simulink library "vehicle_model"  (R2020b)
settings: Solver=ode45  StartTime=0.0  StopTime=10.0  RelTol=1e-3  EnableMultiTasking=on
undefined symbols (not defined in the file): DiscIntNeverNeededParam, par_VEH, select_To_Wks_akt, stepsize, v0
libraries: $bdroot x8, pacejka_trans x6, simulink x4, body_chassis_vert x1
(part 4 of 4)

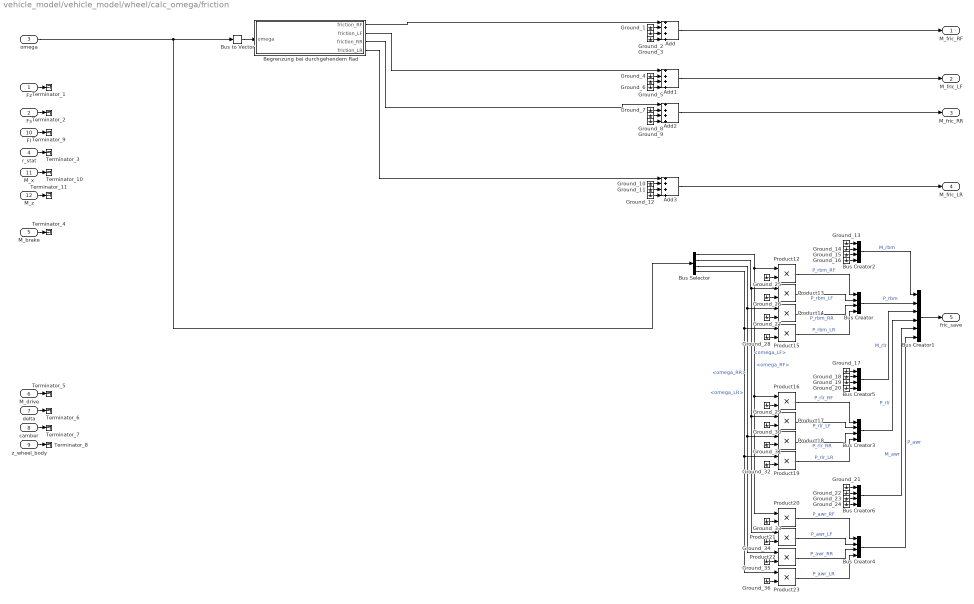
== system vehicle_model/vehicle_model/wheel/calc_omega/friction ==
  Fz : Inport
  Fs : Inport  Port=2
  omega : Inport  Port=3
  r_stat : Inport  Port=4
  M_brake : Inport  Port=5
  M_drive : Inport  Port=6
  delta : Inport  Port=7
  camber : Inport  Port=8
  z_wheel_body : Inport  Port=9
  Fl : Inport  Port=10
  M_x : Inport  Port=11
  M_z : Inport  Port=12
  Add{,1..3} (4 alike) : Sum  Inputs=++++
  Begrenzung bei durchgehendem Rad : Subsystem
  Bus Creator{,2..6} (6 alike) : BusCreator  Inputs=4
  Bus Creator1 : BusCreator  Inputs=6
  Bus Selector : BusSelector  OutputSignals=omega_RF,omega_LF,omega_RR,omega_LR
  Bus to Vector : BusToVector
  Ground_{1..36} (36 alike) : Ground
  Product{12..23} (12 alike) : Product
  Terminator_{1..11} (11 alike) : Terminator
  M_fric_RF : Outport  VectorParamsAs1DForOutWhenUnconnected=off
  M_fric_LF : Outport  Port=2  VectorParamsAs1DForOutWhenUnconnected=off
  M_fric_RR : Outport  Port=3  VectorParamsAs1DForOutWhenUnconnected=off
  M_fric_LR : Outport  Port=4  VectorParamsAs1DForOutWhenUnconnected=off
  fric_save : Outport  Port=5  VectorParamsAs1DForOutWhenUnconnected=off
  wires:
  Ground_36/1 -> Product23/2
  Ground_35/1 -> Product22/2
  Ground_34/1 -> Product21/2
  Ground_33/1 -> Product20/2
  Ground_32/1 -> Product19/2
  Ground_31/1 -> Product18/2
  Ground_30/1 -> Product17/2
  Ground_29/1 -> Product16/2
  Ground_28/1 -> Product15/2
  Ground_27/1 -> Product14/2
  Ground_26/1 -> Product13/2
  Ground_25/1 -> Product12/2
  Ground_24/1 -> Bus Creator6/4
  Ground_23/1 -> Bus Creator6/3
  Ground_22/1 -> Bus Creator6/2
  Ground_21/1 -> Bus Creator6/1
  Ground_20/1 -> Bus Creator5/4
  Ground_19/1 -> Bus Creator5/3
  Ground_18/1 -> Bus Creator5/2
  Ground_17/1 -> Bus Creator5/1
  Ground_16/1 -> Bus Creator2/4
  Ground_15/1 -> Bus Creator2/3
  Ground_14/1 -> Bus Creator2/2
  Ground_13/1 -> Bus Creator2/1
  Ground_12/1 -> Add3/4
  Ground_11/1 -> Add3/3
  Ground_10/1 -> Add3/2
  Ground_9/1 -> Add2/4
  Ground_8/1 -> Add2/3
  Ground_7/1 -> Add2/2
  Ground_6/1 -> Add1/4
  Ground_5/1 -> Add1/3
  Ground_4/1 -> Add1/2
  Ground_3/1 -> Add/4
  Ground_2/1 -> Add/3
  Ground_1/1 -> Add/2
  M_z/1 -> Terminator_11/1
  M_x/1 -> Terminator_10/1
  Fl/1 -> Terminator_9/1
  z_wheel_body/1 -> Terminator_8/1
  camber/1 -> Terminator_7/1
  delta/1 -> Terminator_6/1
  M_drive/1 -> Terminator_5/1
  M_brake/1 -> Terminator_4/1
  r_stat/1 -> Terminator_3/1
  Fs/1 -> Terminator_2/1
  Fz/1 -> Terminator_1/1
  Bus to Vector/1 -> Begrenzung bei durchgehendem Rad/1(omega)
  omega/1 -> Bus Selector/1, Bus to Vector/1
  Begrenzung bei durchgehendem Rad/1(friction_RF) -> Add/1
  Begrenzung bei durchgehendem Rad/2(friction_LF) -> Add1/1
  Begrenzung bei durchgehendem Rad/3(friction_RR) -> Add2/1
  Begrenzung bei durchgehendem Rad/4(friction_LR) -> Add3/1
  Add/1 -> M_fric_RF/1
  Add1/1 -> M_fric_LF/1
  Add2/1 -> M_fric_RR/1
  Add3/1 -> M_fric_LR/1
  Bus Selector/1 -> Product12/1, Product20/1, Product16/1  "<omega_RF>"
  Bus Selector/2 -> Product21/1, Product17/1, Product13/1  "<omega_LF>"
  Bus Selector/3 -> Product22/1, Product18/1, Product14/1  "<omega_RR>"
  Bus Selector/4 -> Product23/1, Product19/1, Product15/1  "<omega_LR>"
  Product12/1 -> Bus Creator/1  "P_rbm_RF"
  Product13/1 -> Bus Creator/2  "P_rbm_LF"
  Product14/1 -> Bus Creator/3  "P_rbm_RR"
  Product15/1 -> Bus Creator/4  "P_rbm_LR"
  Bus Creator/1 -> Bus Creator1/2  "P_rbm"
  Bus Creator2/1 -> Bus Creator1/1  "M_rbm"
  Bus Creator1/1 -> fric_save/1
  Product16/1 -> Bus Creator3/1  "P_rlr_RF"
  Product17/1 -> Bus Creator3/2  "P_rlr_LF"
  Product18/1 -> Bus Creator3/3  "P_rlr_RR"
  Product19/1 -> Bus Creator3/4  "P_rlr_LR"
  Bus Creator5/1 -> Bus Creator1/3  "M_rlr"
  Bus Creator3/1 -> Bus Creator1/4  "P_rlr"
  Product20/1 -> Bus Creator4/1  "P_awr_RF"
  Product21/1 -> Bus Creator4/2  "P_awr_LF"
  Product22/1 -> Bus Creator4/3  "P_awr_RR"
  Product23/1 -> Bus Creator4/4  "P_awr_LR"
  Bus Creator6/1 -> Bus Creator1/5  "M_awr"
  Bus Creator4/1 -> Bus Creator1/6  "P_awr"

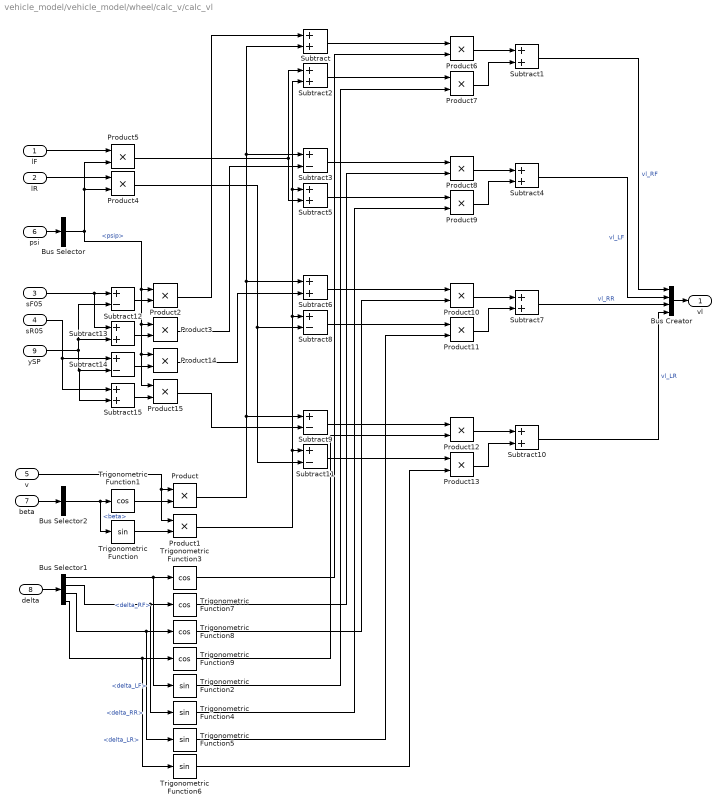
== system vehicle_model/vehicle_model/wheel/calc_v/calc_vl ==
  lF : Inport
  lR : Inport  Port=2
  sF05 : Inport  Port=3
  sR05 : Inport  Port=4
  v : Inport  Port=5
  psi : Inport  Port=6
  beta : Inport  Port=7
  delta : Inport  Port=8
  ySP : Inport  Port=9
  Bus Creator : BusCreator  Inputs=4
  Bus Selector : BusSelector  OutputSignals=psip
  Bus Selector1 : BusSelector  OutputSignals=delta_RF,delta_LF,delta_RR,delta_LR
  Bus Selector2 : BusSelector  OutputSignals=beta
  Product{,1..15} (16 alike) : Product  RndMeth=Zero
  Subtract{,1..2,4..7,10,13,15} (10 alike) : Sum
  Subtract{3,8..9,11..12,14} (6 alike) : Sum  Inputs=+-
  Trigonometric Function{,2,4..6} (5 alike) : Trigonometry
  Trigonometric Function{1,3,7..9} (5 alike) : Trigonometry  Operator=cos
  vl : Outport  VectorParamsAs1DForOutWhenUnconnected=off
  wires:
  Subtract1/1 -> Bus Creator/1  "vl_RF"
  Subtract4/1 -> Bus Creator/2  "vl_LF"
  Subtract7/1 -> Bus Creator/3  "vl_RR"
  Subtract10/1 -> Bus Creator/4  "vl_LR"
  Bus Creator/1 -> vl/1
  psi/1 -> Bus Selector/1
  delta/1 -> Bus Selector1/1
  beta/1 -> Bus Selector2/1
  Bus Selector2/1 -> Trigonometric Function1/1, Trigonometric Function/1  "<beta>"
  v/1 -> Product/1, Product1/1
  Trigonometric Function1/1 -> Product/2
  Trigonometric Function/1 -> Product1/2
  Bus Selector/1 -> Product4/2, Product5/2, Product15/1, Product14/1, Product3/1, Product2/1  "<psip>"
  lF/1 -> Product5/1
  lR/1 -> Product4/1
  Bus Selector1/1 -> Trigonometric Function2/1, Trigonometric Function3/1  "<delta_RF>"
  Bus Selector1/2 -> Trigonometric Function4/1, Trigonometric Function7/1  "<delta_LF>"
  Bus Selector1/3 -> Trigonometric Function5/1, Trigonometric Function8/1  "<delta_RR>"
  Bus Selector1/4 -> Trigonometric Function6/1, Trigonometric Function9/1  "<delta_LR>"
  Product/1 -> Subtract/2, Subtract3/1, Subtract6/1, Subtract9/1
  Subtract/1 -> Product6/1
  Trigonometric Function3/1 -> Product6/2
  Product6/1 -> Subtract1/1
  Product7/1 -> Subtract1/2
  Trigonometric Function2/1 -> Product7/2
  Subtract2/1 -> Product7/1
  Product1/1 -> Subtract2/2, Subtract5/1, Subtract8/1, Subtract11/1
  Product5/1 -> Subtract2/1, Subtract5/2
  Subtract3/1 -> Product8/1
  Product8/1 -> Subtract4/1
  Product9/1 -> Subtract4/2
  Subtract5/1 -> Product9/1
  Trigonometric Function7/1 -> Product8/2
  Trigonometric Function4/1 -> Product9/2
  Subtract6/1 -> Product10/1
  Product10/1 -> Subtract7/1
  Product11/1 -> Subtract7/2
  Subtract8/1 -> Product11/1
  Trigonometric Function8/1 -> Product10/2
  Trigonometric Function5/1 -> Product11/2
  Product4/1 -> Subtract8/2, Subtract11/2
  Subtract9/1 -> Product12/1
  Product12/1 -> Subtract10/1
  Product13/1 -> Subtract10/2
  Subtract11/1 -> Product13/1
  Trigonometric Function9/1 -> Product12/2
  Trigonometric Function6/1 -> Product13/2
  sF05/1 -> Subtract13/1, Subtract12/1
  ySP/1 -> Subtract13/2, Subtract12/2, Subtract15/2, Subtract14/2
  sR05/1 -> Subtract15/1, Subtract14/1
  Subtract15/1 -> Product15/2
  Subtract14/1 -> Product14/2
  Subtract13/1 -> Product3/2
  Subtract12/1 -> Product2/2
  Product2/1 -> Subtract/1
  Product3/1 -> Subtract3/2
  Product14/1 -> Subtract6/2
  Product15/1 -> Subtract9/2

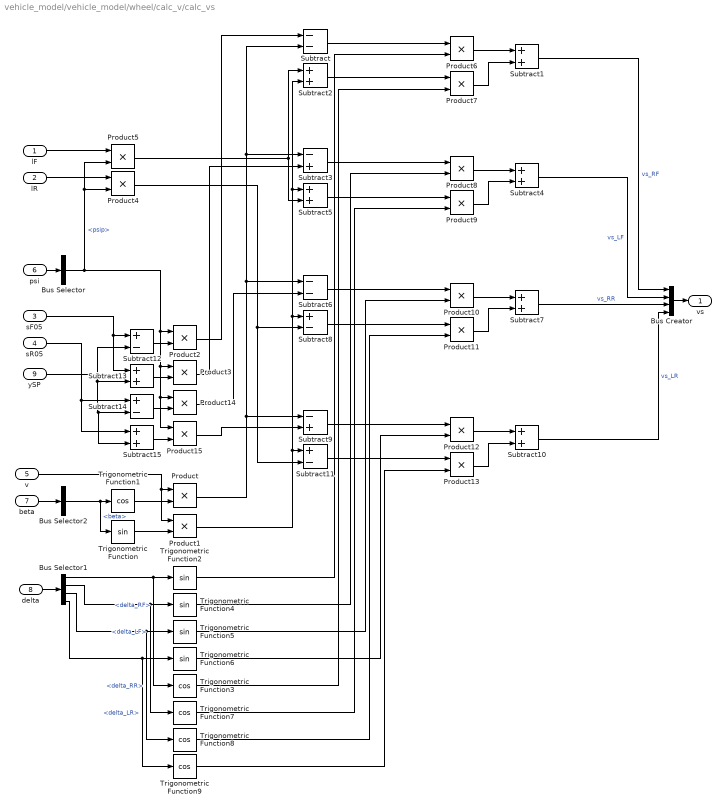
== system vehicle_model/vehicle_model/wheel/calc_v/calc_vs ==
  lF : Inport
  lR : Inport  Port=2
  sF05 : Inport  Port=3
  sR05 : Inport  Port=4
  v : Inport  Port=5
  psi : Inport  Port=6
  beta : Inport  Port=7
  delta : Inport  Port=8
  ySP : Inport  Port=9
  Bus Creator : BusCreator  Inputs=4
  Bus Selector : BusSelector  OutputSignals=psip
  Bus Selector1 : BusSelector  OutputSignals=delta_RF,delta_LF,delta_RR,delta_LR
  Bus Selector2 : BusSelector  OutputSignals=beta
  Product{,1..15} (16 alike) : Product  RndMeth=Zero
  Subtract : Sum  Inputs=--
  Subtract{1..2,4..5,7,10,13,15} (8 alike) : Sum
  Subtract{8,11..12,14} (4 alike) : Sum  Inputs=+-
  Subtract3 : Sum  Inputs=-+
  Subtract6 : Sum  Inputs=--
  Subtract9 : Sum  Inputs=-+
  Trigonometric Function{,2,4..6} (5 alike) : Trigonometry
  Trigonometric Function{1,3,7..9} (5 alike) : Trigonometry  Operator=cos
  vs : Outport  VectorParamsAs1DForOutWhenUnconnected=off
  wires:
  Trigonometric Function9/1 -> Product13/2
  Trigonometric Function6/1 -> Product12/2
  Subtract11/1 -> Product13/1
  Product13/1 -> Subtract10/2
  Product12/1 -> Subtract10/1
  Subtract9/1 -> Product12/1
  Product4/1 -> Subtract11/2, Subtract8/2
  Trigonometric Function8/1 -> Product11/2
  Trigonometric Function5/1 -> Product10/2
  Subtract8/1 -> Product11/1
  Product11/1 -> Subtract7/2
  Product10/1 -> Subtract7/1
  Subtract6/1 -> Product10/1
  Trigonometric Function7/1 -> Product9/2
  Trigonometric Function4/1 -> Product8/2
  Subtract5/1 -> Product9/1
  Product9/1 -> Subtract4/2
  Product8/1 -> Subtract4/1
  Subtract3/1 -> Product8/1
  Product5/1 -> Subtract5/2, Subtract2/1
  Product1/1 -> Subtract11/1, Subtract8/1, Subtract5/1, Subtract2/2
  Subtract2/1 -> Product7/1
  Trigonometric Function3/1 -> Product7/2
  Product7/1 -> Subtract1/2
  Product6/1 -> Subtract1/1
  Trigonometric Function2/1 -> Product6/2
  Subtract/1 -> Product6/1
  Product/1 -> Subtract9/1, Subtract6/1, Subtract3/1, Subtract/2
  Bus Selector1/4 -> Trigonometric Function9/1, Trigonometric Function6/1  "<delta_LR>"
  Bus Selector1/3 -> Trigonometric Function8/1, Trigonometric Function5/1  "<delta_RR>"
  Bus Selector1/2 -> Trigonometric Function7/1, Trigonometric Function4/1  "<delta_LF>"
  Bus Selector1/1 -> Trigonometric Function3/1, Trigonometric Function2/1  "<delta_RF>"
  lR/1 -> Product4/1
  lF/1 -> Product5/1
  Trigonometric Function/1 -> Product1/2
  Trigonometric Function1/1 -> Product/2
  v/1 -> Product1/1, Product/1
  Bus Selector2/1 -> Trigonometric Function/1, Trigonometric Function1/1  "<beta>"
  beta/1 -> Bus Selector2/1
  delta/1 -> Bus Selector1/1
  psi/1 -> Bus Selector/1
  Bus Creator/1 -> vs/1
  Subtract10/1 -> Bus Creator/4  "vs_LR"
  Subtract7/1 -> Bus Creator/3  "vs_RR"
  Subtract4/1 -> Bus Creator/2  "vs_LF"
  Subtract1/1 -> Bus Creator/1  "vs_RF"
  Bus Selector/1 -> Product15/1, Product14/1, Product3/1, Product2/1, Product5/2, Product4/2  "<psip>"
  sF05/1 -> Subtract13/1, Subtract12/1
  ySP/1 -> Subtract15/2, Subtract14/2, Subtract13/2, Subtract12/2
  sR05/1 -> Subtract15/1, Subtract14/1
  Subtract15/1 -> Product15/2
  Subtract14/1 -> Product14/2
  Subtract13/1 -> Product3/2
  Subtract12/1 -> Product2/2
  Product2/1 -> Subtract/1
  Product3/1 -> Subtract3/2
  Product14/1 -> Subtract6/2
  Product15/1 -> Subtract9/2

== system vehicle_model/vehicle_model/wheel/v0_korr/Subsystem4 ==
  vl : Inport
  v_low : Inport  Port=2
  r_dyn : Inport  Port=3
  omega : Inport  Port=4
  Abs : Abs
  Constant1 : Constant
  Constant2 : Constant  Value=pi
  Constant3 : Constant  Value=0.5
  Constant4 : Constant  Value=0  VectorParams1D=off
  Constant5 : Constant
  Divide1 : Product  Inputs=*/
  Divide2 : Product  Inputs=*/
  Divide{3..6} (4 alike) : Product  Inputs=**
  Gain : Gain  Gain=2
  Saturation Dynamic : simulink/Discontinuities/Saturation Dynamic  OutMin=[]  OutMax=[]  OutDataTypeStr=Inherit: Same as second input  OutDataType=fixdt(1, 16)  OutScaling=2^-10  DoSatur=off
  Saturation Dynamic1 : simulink/Discontinuities/Saturation Dynamic  OutMin=[]  OutMax=[]  OutDataTypeStr=Inherit: Same as second input  OutDataType=fixdt(1, 16)  OutScaling=2^-10  DoSatur=off
  Subtract : Sum  Inputs=+-
  Subtract1 : Sum
  Subtract2 : Sum  Inputs=-+
  Subtract3 : Sum  Inputs=+-
  Subtract5 : Sum
  Switch : Switch  Threshold=-0.0001
  Trigonometric Function : Trigonometry  Operator=cos
  omega_out : Outport  VectorParamsAs1DForOutWhenUnconnected=off
  wires:
  Gain/1 -> Saturation Dynamic1/1
  Saturation Dynamic1/1 -> Subtract3/1
  Subtract3/1 -> Divide2/1
  Subtract2/1 -> Divide6/1
  Divide5/1 -> Subtract5/1
  Switch/1 -> Subtract2/1, Divide5/1
  Constant5/1 -> Subtract2/2, Switch/3
  Divide4/1 -> Switch/1
  Divide6/1 -> Subtract5/2
  Subtract5/1 -> omega_out/1
  omega/1 -> Divide6/2
  Constant4/1 -> Saturation Dynamic/3, Saturation Dynamic1/3
  Saturation Dynamic/1 -> Subtract/1
  Abs/1 -> Saturation Dynamic1/2, Saturation Dynamic/2
  Constant3/1 -> Divide4/2
  Subtract1/1 -> Divide4/1
  Constant1/1 -> Subtract1/2
  Trigonometric Function/1 -> Subtract1/1
  Divide3/1 -> Trigonometric Function/1
  Constant2/1 -> Divide3/2
  Divide2/1 -> Divide3/1
  Subtract/1 -> Switch/2
  r_dyn/1 -> Divide1/2
  v_low/1 -> Gain/1, Saturation Dynamic/1, Divide2/2, Subtract3/2, Subtract/2
  Divide1/1 -> Divide5/2
  vl/1 -> Divide1/1, Abs/1

== system vehicle_model/vehicle_model/wheel/wheel_lift/wheel_lift_RF ==
  Fz_tire_wheel : Inport
  Fzt : Inport  Port=2
  z_init : Inport  Port=3
  Add : Sum  Inputs=+-
  Bus Creator : BusCreator  Inputs=3
  Discrete-Time Integrator : DiscreteIntegrator  ExternalReset=level  SampleTime=-1  ICPrevOutput=DiscIntNeverNeededParam  ICPrevScaledInput=DiscIntNeverNeededParam
  Discrete-Time Integrator1 : DiscreteIntegrator  ExternalReset=level  InitialConditionSource=external  SampleTime=-1  ICPrevOutput=DiscIntNeverNeededParam  ICPrevScaledInput=DiscIntNeverNeededParam
  Divide : Product  Inputs=*/
  Gain : Gain  Gain=0.5
  zwheel : Outport  VectorParamsAs1DForOutWhenUnconnected=off
  wires:
  Add/1 -> Divide/1
  Fz_tire_wheel/1 -> Add/1
  Fzt/1 -> Add/2
  Divide/1 -> Discrete-Time Integrator/1, Bus Creator/3  "zwheelpp"
  Discrete-Time Integrator/1 -> Discrete-Time Integrator1/1, Bus Creator/2  "zwheelp"
  Discrete-Time Integrator1/1 -> Bus Creator/1  "zwheel"
  Bus Creator/1 -> zwheel/1
  [m_usF] -> Gain/1
  Gain/1 -> Divide/2
  [reset] -> Discrete-Time Integrator/2, Discrete-Time Integrator1/2
  z_init/1 -> Discrete-Time Integrator1/3

== system vehicle_model/vehicle_model/wheel/wheel_lift/wheel_lift_RR ==
  Fz_tire_wheel : Inport
  Fzt : Inport  Port=2
  z_init : Inport  Port=3
  Add : Sum  Inputs=+-
  Bus Creator : BusCreator  Inputs=3
  Discrete-Time Integrator : DiscreteIntegrator  ExternalReset=level  SampleTime=-1  ICPrevOutput=DiscIntNeverNeededParam  ICPrevScaledInput=DiscIntNeverNeededParam
  Discrete-Time Integrator1 : DiscreteIntegrator  ExternalReset=level  InitialConditionSource=external  SampleTime=-1  ICPrevOutput=DiscIntNeverNeededParam  ICPrevScaledInput=DiscIntNeverNeededParam
  Divide : Product  Inputs=*/
  Gain : Gain  Gain=0.5
  zwheel : Outport  VectorParamsAs1DForOutWhenUnconnected=off
  wires:
  Add/1 -> Divide/1
  Fz_tire_wheel/1 -> Add/1
  Fzt/1 -> Add/2
  Divide/1 -> Discrete-Time Integrator/1, Bus Creator/3  "zwheelpp"
  Discrete-Time Integrator/1 -> Discrete-Time Integrator1/1, Bus Creator/2  "zwheelp"
  Discrete-Time Integrator1/1 -> Bus Creator/1  "zwheel"
  Bus Creator/1 -> zwheel/1
  [m_usR] -> Gain/1
  Gain/1 -> Divide/2
  [reset] -> Discrete-Time Integrator/2, Discrete-Time Integrator1/2
  z_init/1 -> Discrete-Time Integrator1/3

== system vehicle_model/simplified_vehicle_model/body_chassis_vert/suspension/damper/Front ==
  z_pitchp : Inport
  z_vertp : Inport  Port=2
  z_wheel_vertp : Inport  Port=3
  Add : Sum  Inputs=++-
  Divide : Product  Inputs=*/
  Product1 : Product  RndMeth=Zero
  Product2 : Product  RndMeth=Zero
  Product3 : Product  RndMeth=Zero
  Switch : Switch
  compression : Polyval  Coefs=par_VEH.ddF_comp
  rebound : Polyval  Coefs=par_VEH.ddF_reb
  Fz_damper : Outport  VectorParamsAs1DForOutWhenUnconnected=off
  P_damper : Outport  Port=2  VectorParamsAs1DForOutWhenUnconnected=off
  wires:
  Product1/1 -> P_damper/1
  z_wheel_vertp/1 -> Add/3
  z_pitchp/1 -> Add/1
  z_vertp/1 -> Add/2
  [sdF] -> Divide/1
  [sF] -> Divide/2
  Divide/1 -> Product2/2, Product3/2
  Product2/1 -> Fz_damper/1
  compression/1 -> Switch/3
  rebound/1 -> Switch/1
  Switch/1 -> Product2/1, Product1/1
  Add/1 -> Product3/1
  Product3/1 -> Product1/2, compression/1, Switch/2, rebound/1

== system vehicle_model/simplified_vehicle_model/body_chassis_vert/suspension/damper/Rear ==
  z_pitchp : Inport
  z_vertp : Inport  Port=2
  z_wheel_vertp : Inport  Port=3
  Add : Sum  Inputs=++-
  Divide : Product  Inputs=*/
  Product1 : Product  RndMeth=Zero
  Product2 : Product  RndMeth=Zero
  Product3 : Product  RndMeth=Zero
  Switch : Switch
  compression : Polyval  Coefs=par_VEH.ddR_comp
  rebound : Polyval  Coefs=par_VEH.ddR_reb
  Fz_damper : Outport  VectorParamsAs1DForOutWhenUnconnected=off
  P_damper : Outport  Port=2  VectorParamsAs1DForOutWhenUnconnected=off
  wires:
  Product1/1 -> P_damper/1
  Product3/1 -> compression/1, Product1/2, rebound/1, Switch/2
  Switch/1 -> Product2/1, Product1/1
  z_wheel_vertp/1 -> Add/3
  z_pitchp/1 -> Add/1
  z_vertp/1 -> Add/2
  [sdR] -> Divide/1
  [sR] -> Divide/2
  Divide/1 -> Product3/2, Product2/2
  Product2/1 -> Fz_damper/1
  compression/1 -> Switch/3
  rebound/1 -> Switch/1
  Add/1 -> Product3/1

== system vehicle_model/simplified_vehicle_model/body_chassis_vert/suspension/spring/Front ==
  z_pitch : Inport
  z_vert : Inport  Port=2
  z_wheel_vert : Inport  Port=3
  Add : Sum  Inputs=--+
  Divide : Product  Inputs=*/
  Product : Product
  Product1 : Product
  csRF : Lookup_n-D  NumberOfTableDimensions=1  BreakpointsForDimension1=par_VEH.cF_front(:,1)  Table=par_VEH.cF_front(:,2)  InternalRulePriority=Speed  RndMeth=Simplest  InputSameDT=on
  Fz_spring : Outport  VectorParamsAs1DForOutWhenUnconnected=off
  z_wheel : Outport  Port=2  VectorParamsAs1DForOutWhenUnconnected=off
  wires:
  Product1/1 -> Fz_spring/1
  Add/1 -> Product/1, z_wheel/1
  z_pitch/1 -> Add/1
  z_vert/1 -> Add/2
  z_wheel_vert/1 -> Add/3
  [ssF] -> Divide/1
  [sF] -> Divide/2
  Product/1 -> csRF/1
  Divide/1 -> Product1/2, Product/2
  csRF/1 -> Product1/1

== system vehicle_model/simplified_vehicle_model/body_chassis_vert/suspension/spring/Rear ==
  z_pitch : Inport
  z_vert : Inport  Port=2
  z_wheel_vert : Inport  Port=3
  Add : Sum  Inputs=--+
  Divide : Product  Inputs=*/
  Product : Product
  Product1 : Product
  csRF : Lookup_n-D  NumberOfTableDimensions=1  BreakpointsForDimension1=par_VEH.cF_rear(:,1)  Table=par_VEH.cF_rear(:,2)  InternalRulePriority=Speed  RndMeth=Simplest  InputSameDT=on
  Fz_spring : Outport  VectorParamsAs1DForOutWhenUnconnected=off
  z_wheel : Outport  Port=2  VectorParamsAs1DForOutWhenUnconnected=off
  wires:
  csRF/1 -> Product1/1
  Add/1 -> Product/1, z_wheel/1
  z_pitch/1 -> Add/1
  z_vert/1 -> Add/2
  z_wheel_vert/1 -> Add/3
  [ssR] -> Divide/1
  [sR] -> Divide/2
  Divide/1 -> Product1/2, Product/2
  Product/1 -> csRF/1
  Product1/1 -> Fz_spring/1

== system vehicle_model/simplified_vehicle_model/wheel/calc_omega/friction/Begrenzung bei durchgehendem Rad ==
  omega : Inport
  Abs : Abs
  Bias : Bias  Bias=-350
  Bias1 : Bias  Bias=0.5
  Demux : Demux  Outputs=2
  Gain : Gain  Gain=1000
  Gain1 : Gain  Gain=0.5
  Gain2 : Gain  Gain=1/30
  Product : Product  RndMeth=Zero
  Sign : Signum
  Trigonometric Function : Trigonometry  Operator=tanh
  friction_F : Outport  VectorParamsAs1DForOutWhenUnconnected=off
  friction_R : Outport  Port=2  VectorParamsAs1DForOutWhenUnconnected=off
  wires:
  Gain/1 -> Product/1
  Demux/2 -> friction_R/1
  Demux/1 -> friction_F/1
  Product/1 -> Demux/1
  Sign/1 -> Product/2
  Bias1/1 -> Gain/1
  Gain2/1 -> Trigonometric Function/1
  Bias/1 -> Gain2/1
  Abs/1 -> Bias/1
  omega/1 -> Sign/1, Abs/1
  Trigonometric Function/1 -> Gain1/1
  Gain1/1 -> Bias1/1

== system vehicle_model/vehicle_model/wheel/calc_omega/friction/Begrenzung bei durchgehendem Rad ==
  omega : Inport
  Abs : Abs
  Bias : Bias  Bias=-350
  Bias1 : Bias  Bias=0.5
  Demux : Demux
  Gain : Gain  Gain=1000
  Gain1 : Gain  Gain=0.5
  Gain2 : Gain  Gain=1/30
  Product : Product  RndMeth=Zero
  Sign : Signum
  Trigonometric Function : Trigonometry  Operator=tanh
  friction_RF : Outport  VectorParamsAs1DForOutWhenUnconnected=off
  friction_LF : Outport  Port=2  VectorParamsAs1DForOutWhenUnconnected=off
  friction_RR : Outport  Port=3  VectorParamsAs1DForOutWhenUnconnected=off
  friction_LR : Outport  Port=4  VectorParamsAs1DForOutWhenUnconnected=off
  wires:
  Gain1/1 -> Bias1/1
  Trigonometric Function/1 -> Gain1/1
  omega/1 -> Abs/1, Sign/1
  Abs/1 -> Bias/1
  Bias/1 -> Gain2/1
  Gain2/1 -> Trigonometric Function/1
  Bias1/1 -> Gain/1
  Sign/1 -> Product/2
  Product/1 -> Demux/1
  Demux/1 -> friction_RF/1
  Demux/2 -> friction_LF/1
  Demux/3 -> friction_RR/1
  Demux/4 -> friction_LR/1
  Gain/1 -> Product/1
